simulink model "rfdc_V0_1"  (R2018a)
settings: Solver=VariableStepAuto  StartTime=0.0  StopTime=10.0  RelTol=1e-3
libraries: xbsIndex_r4 x10
settings Model: Creator=wei  LastModifiedBy=wei

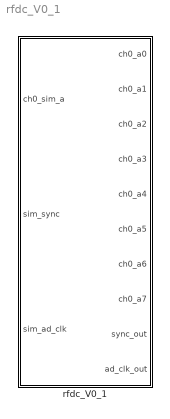
== system rfdc_V0_1 ==
  rfdc_V0_1 : Subsystem  Tag=xps:rfdc_V0_1  mask(rfdc){f_sample=2048}
      mask prompts: f_sample "ADC Clock Rate(Mhz)"
      mask init:
      | rfdc_v0_1_init(gcb)

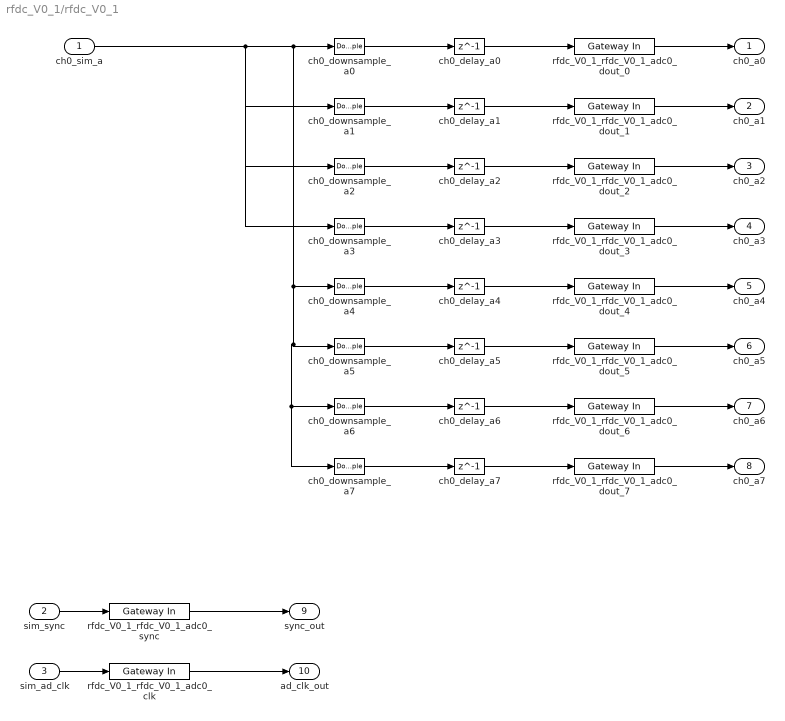
== system rfdc_V0_1/rfdc_V0_1 ==
  ch0_sim_a : Inport
  sim_sync : Inport  Port=2
  sim_ad_clk : Inport  Port=3
  ch0_delay_a{0..7} (8 alike) : Delay  DelayLength=1  InitialCondition=0  InputProcessing=Inherited
  ch0_downsample_a0 : DownSample  N=8  RateOptions=Allow multirate processing
  ch0_downsample_a1 : DownSample  N=8  phase=1  RateOptions=Allow multirate processing
  ch0_downsample_a2 : DownSample  N=8  phase=2  RateOptions=Allow multirate processing
  ch0_downsample_a3 : DownSample  N=8  phase=3  RateOptions=Allow multirate processing
  ch0_downsample_a4 : DownSample  N=8  phase=4  RateOptions=Allow multirate processing
  ch0_downsample_a5 : DownSample  N=8  phase=5  RateOptions=Allow multirate processing
  ch0_downsample_a6 : DownSample  N=8  phase=6  RateOptions=Allow multirate processing
  ch0_downsample_a7 : DownSample  N=8  phase=7  RateOptions=Allow multirate processing
  rfdc_V0_1_rfdc_V0_1_adc0_clk : xbsIndex_r4/Gateway In  gui_display_data_type=Boolean  arith_type=Boolean  n_bits=16  bin_pt=14  preci_type=Single  exp_width=8  frac_width=24  rows=1  columns=1  quantization="Round  (unbiased: +/- Inf)"  overflow=Saturate  period=1  UseAsADC=off  ADCChannel='1'  interface=None  automatic_assignment=on  address_offset=hex2dec('00')  intf_name=''  intf_description=''  default_value=0  timing_constraint=None  locs_specified=off  LOCs={}  io_standard={}  inherit_from_input=off  hdl_port=on  dbl_ovrd=off  block_type=gatewayin
  rfdc_V0_1_rfdc_V0_1_adc0_dout_{0..7} (8 alike) : xbsIndex_r4/Gateway In  gui_display_data_type=Fixed-point  arith_type=Unsigned  n_bits=16  bin_pt=0  preci_type=Single  exp_width=8  frac_width=24  rows=1  columns=1  quantization=Truncate  overflow=Wrap  period=1  UseAsADC=off  ADCChannel='1'  interface=None  automatic_assignment=on  address_offset=hex2dec('00')  intf_name=''  intf_description=''  default_value=0  timing_constraint=None  locs_specified=off  LOCs={}  io_standard={}  inherit_from_input=off  hdl_port=on  dbl_ovrd=off  block_type=gatewayin
  rfdc_V0_1_rfdc_V0_1_adc0_sync : xbsIndex_r4/Gateway In  gui_display_data_type=Boolean  arith_type=Boolean  n_bits=16  bin_pt=14  preci_type=Single  exp_width=8  frac_width=24  rows=1  columns=1  quantization="Round  (unbiased: +/- Inf)"  overflow=Saturate  period=1  UseAsADC=off  ADCChannel='1'  interface=None  automatic_assignment=on  address_offset=hex2dec('00')  intf_name=''  intf_description=''  default_value=0  timing_constraint=None  locs_specified=off  LOCs={}  io_standard={}  inherit_from_input=off  hdl_port=on  dbl_ovrd=off  block_type=gatewayin
  ch0_a0 : Outport
  ch0_a1 : Outport  Port=2
  ch0_a2 : Outport  Port=3
  ch0_a3 : Outport  Port=4
  ch0_a4 : Outport  Port=5
  ch0_a5 : Outport  Port=6
  ch0_a6 : Outport  Port=7
  ch0_a7 : Outport  Port=8
  sync_out : Outport  Port=9
  ad_clk_out : Outport  Port=10
  wires:
  ch0_downsample_a0/1 -> ch0_delay_a0/1
  ch0_delay_a0/1 -> rfdc_V0_1_rfdc_V0_1_adc0_dout_0/1
  rfdc_V0_1_rfdc_V0_1_adc0_dout_0/1 -> ch0_a0/1
  ch0_downsample_a1/1 -> ch0_delay_a1/1
  ch0_delay_a1/1 -> rfdc_V0_1_rfdc_V0_1_adc0_dout_1/1
  rfdc_V0_1_rfdc_V0_1_adc0_dout_1/1 -> ch0_a1/1
  ch0_downsample_a2/1 -> ch0_delay_a2/1
  ch0_delay_a2/1 -> rfdc_V0_1_rfdc_V0_1_adc0_dout_2/1
  rfdc_V0_1_rfdc_V0_1_adc0_dout_2/1 -> ch0_a2/1
  ch0_downsample_a3/1 -> ch0_delay_a3/1
  ch0_delay_a3/1 -> rfdc_V0_1_rfdc_V0_1_adc0_dout_3/1
  rfdc_V0_1_rfdc_V0_1_adc0_dout_3/1 -> ch0_a3/1
  sim_sync/1 -> rfdc_V0_1_rfdc_V0_1_adc0_sync/1
  rfdc_V0_1_rfdc_V0_1_adc0_sync/1 -> sync_out/1
  sim_ad_clk/1 -> rfdc_V0_1_rfdc_V0_1_adc0_clk/1
  rfdc_V0_1_rfdc_V0_1_adc0_clk/1 -> ad_clk_out/1
  ch0_delay_a5/1 -> rfdc_V0_1_rfdc_V0_1_adc0_dout_5/1
  ch0_downsample_a6/1 -> ch0_delay_a6/1
  rfdc_V0_1_rfdc_V0_1_adc0_dout_7/1 -> ch0_a7/1
  ch0_delay_a7/1 -> rfdc_V0_1_rfdc_V0_1_adc0_dout_7/1
  ch0_delay_a6/1 -> rfdc_V0_1_rfdc_V0_1_adc0_dout_6/1
  rfdc_V0_1_rfdc_V0_1_adc0_dout_6/1 -> ch0_a6/1
  ch0_delay_a4/1 -> rfdc_V0_1_rfdc_V0_1_adc0_dout_4/1
  rfdc_V0_1_rfdc_V0_1_adc0_dout_4/1 -> ch0_a4/1
  rfdc_V0_1_rfdc_V0_1_adc0_dout_5/1 -> ch0_a5/1
  ch0_downsample_a7/1 -> ch0_delay_a7/1
  ch0_downsample_a5/1 -> ch0_delay_a5/1
  ch0_downsample_a4/1 -> ch0_delay_a4/1
  ch0_sim_a/1 -> ch0_downsample_a7/1, ch0_downsample_a6/1, ch0_downsample_a5/1, ch0_downsample_a4/1, ch0_downsample_a0/1, ch0_downsample_a3/1, ch0_downsample_a1/1, ch0_downsample_a2/1
